simulink model "IndustrialMicrogrid"  (R2025a)
settings: Solver=FixedStepAuto  StartTime=0.0  StopTime=8  FixedStep=Ts  RelTol=1e-3
PostLoadFcn:
  | IndustrialMicrogridInputData
  | GfmGridFormingConverterInputParameters
model workspace (MAT data in the model file):
  caseNum = 2
undefined symbols (not defined in the file): base, BESS, DiscIntNeverNeededParam, grid, Grid, gridInverter, machine, microgrid, PV, PVInverter, PVTransformer, scrFactorRg, scrFactorXg, transformer, Transition_and_Dispatch_ControlModeType, Ts
libraries: ee_lib x126, fl_lib x91, eeGeneralControl x73, nesl_utility x50, nesl_utility_internal x46, simulink x30, eeTransforms x11, eeSinusoidalMeasurementV2 x5, eeTotalHarmonicDistorsion x4, slpidlib x3, simulink_extras x2, eePowerMeasurement x2
(part 8 of 12)

== system IndustrialMicrogrid/MG1 Primary Substation/BESS and Controller/BESS/Filter & Sensor ==
  Current Sensor (Three-Phase) : ee_lib/Sensors & Transducers/Current Sensor (Three-Phase)
  Electrical Reference1 : fl_lib/Electrical/Electrical Elements/Electrical Reference
  Low-Pass Filter (Discrete or Continuous)1 : eeGeneralControl/Low-Pass Filter (Discrete or Continuous)  K=1  T=1/(200*gridInverter.frequency)  B=inf  A=-inf  init_option=Specify as parameter  x0=0  Ts=gridInverter.controller.VoltageControlSampleTime
  Low-Pass Filter (Discrete or Continuous)2 : eeGeneralControl/Low-Pass Filter (Discrete or Continuous)  K=1  T=1/(200*gridInverter.frequency)  B=inf  A=-inf  init_option=Specify as parameter  x0=0  Ts=gridInverter.controller.VoltageControlSampleTime
  Neutral Port (Three-Phase) : ee_lib/Connectors & References/Neutral Port (Three-Phase)  G_parasitic=1e-12 1/Ohm
      settings: InternalSimscapePortConfiguration="{\"Bottom\":[],\"Left\":[{\"id\":\"N\",\"label\":\"~\",\"type\":\"foundation.electrical.three_phase\"}],\"Right\":[{\"id\":\"n\",\"label\":\"n\",\"type\":\"foundation.electrical.electrical\"}],\"Top\":[]}"
  PS-Simulink Converter : nesl_utility/PS-Simulink Converter  PhysicalDomain=network_engine_domain  SubClassName=ps_output  LeftPortType=input  RightPortType=output  PseudoPeriodic=off  Frequencies=[]  VectorFormat=inherit  Unit=inherit  AffineConversion=off
  PS-Simulink Converter1 : nesl_utility/PS-Simulink Converter  PhysicalDomain=network_engine_domain  SubClassName=ps_output  LeftPortType=input  RightPortType=output  PseudoPeriodic=off  Frequencies=[]  VectorFormat=inherit  Unit=inherit  AffineConversion=off
  Phase Voltage Sensor (Three-Phase) : ee_lib/Sensors & Transducers/Phase Voltage Sensor (Three-Phase)
  RLC (Three-Phase) : ee_lib/Passive/RLC Assemblies/RLC (Three-Phase)  port_option=ee.enum.threePhasePort.composite  component_structure=ee.enum.rlc.structure.SeriesRL  R=gridInverter.lineResistance Ohm  L=gridInverter.L*10 H  C=1e-6 F  R_parasitic=0 Ohm  G_parasitic=0 1/Ohm  IL_specify=off  IL_priority=High  IL=[0, 0, 0] A  IL_nominal_specify=off  IL_nominal_value=1  IL_nominal_unit=A  VC_specify=off  VC_priority=High  VC=[0, 0, 0] V  VC_nominal_specify=off  VC_nominal_value=1  VC_nominal_unit=V
      settings: InternalSimscapePortConfiguration="{\"Bottom\":[],\"Left\":[{\"id\":\"N1\",\"label\":\"~1\",\"type\":\"foundation.electrical.three_phase\"}],\"Right\":[{\"id\":\"N2\",\"label\":\"~2\",\"type\":\"foundation.electrical.three_phase\"}],\"Top\":[]}"
  Inabc : PMIOPort  Side=Left
  Opabc : PMIOPort  Port=2  Side=Right
  Iabc : Outport
  Vabc : Outport  Port=2
  wires:
  PS-Simulink Converter1/1 -> Low-Pass Filter (Discrete or Continuous)1/1
  Low-Pass Filter (Discrete or Continuous)2/1 -> Iabc/1
  PS-Simulink Converter/1 -> Low-Pass Filter (Discrete or Continuous)2/1
  Low-Pass Filter (Discrete or Continuous)1/1 -> Vabc/1
  connections:
  Electrical Reference1/LConn1 -- Neutral Port (Three-Phase)/RConn1
  PS-Simulink Converter1/LConn1 -- Phase Voltage Sensor (Three-Phase)/RConn1
  Current Sensor (Three-Phase)/RConn2 -- RLC (Three-Phase)/LConn1
  Neutral Port (Three-Phase)/LConn1 -- Phase Voltage Sensor (Three-Phase)/RConn2
  Current Sensor (Three-Phase)/LConn1 -- Inabc/RConn1
  PS-Simulink Converter/LConn1 -- Current Sensor (Three-Phase)/RConn1
  Phase Voltage Sensor (Three-Phase)/LConn1 -- Opabc/RConn1 -- RLC (Three-Phase)/RConn1

== system IndustrialMicrogrid/MG1 Primary Substation/BESS and Controller/BESS/Grid-Forming Converter Control ==
  Pref : Inport
  Qref : Inport  Port=2
  Vref : Inport  Port=3
  Fref : Inport  Port=4
  CntrlFlag : Inport  Port=5
  BlackStart : Inport  Port=6
  Igabc : Inport  Port=7
  Vgabc : Inport  Port=8
  Current Limiting : Subsystem
  Grid Voltage Reactive Power Support : Subsystem
  Measurement : Subsystem
      mask Display: image('$imagefile'); % Use "Edit Image" on toolstrip to change.
  Power Control : Subsystem
  VoltageCurrentControl : Subsystem
      settings: PortSchema="{\"entries\":[{\"content\":{\"sides\":[{\"content\":{\"connectorIds\":[\"In1\",\"In2\",\"In3\"]},\"type\":\"ConnectorPlacement.EquallySpacedRectSide\",\"uuid\":\"0bf15a12-7bc0-47e4-89bd-435769673763\"},{\"content\":{\"connectorIds\":[\"Out1\"],\"side\":\"RIGHT\"},\"type\":\"ConnectorPlacement.EquallySpacedRectSide\",\"uuid\":\"44a15d74-8878-4ec6-abe4-be0b1b609519\"},{\"content\":{\"connectorIds\":[\"In4\"],\"side\":\"TOP\"},\"type\":\"ConnectorPlacement.EquallySpacedRectSide\",\"uuid\":\"7a96781e-5638-4b2a-8101-d5785aae9f0f\"}]},\"type\":\"ConnectorPlacement.EquallySpacedConnector\",\"uuid\":\"4b3373ad-cf20-4175-894e-3bd1604dd0ce\"}],\"packageUris\":[\"http://schema.mathworks.com/mf0/Connector/R2020b\"],\"version\":\"1.0\"}"
  mabc : Outport
  Pmeas : Outport  Port=2
  Qmeas : Outport  Port=3
  fmeas : Outport  Port=4
  wires:
  VoltageCurrentControl/1(mabc) -> mabc/1
  Vgabc/1 -> Measurement/1(Vgabcc)
  Igabc/1 -> Measurement/2(Igabc)
  Measurement/2(Pmeas) -> Pmeas/1
  Measurement/3(Qmeas) -> Qmeas/1
  Measurement/1(measure) -> Current Limiting/1(measure), VoltageCurrentControl/4(measure), Power Control/1(measure), Grid Voltage Reactive Power Support/1(measure)
  Power Control/3(angle) -> Measurement/3(Angle)
  Power Control/1(reactiveControl) -> Current Limiting/2(reactiveControl)
  Power Control/2(activeControl) -> VoltageCurrentControl/2(activeControl)
  Current Limiting/1(currentLimiting) -> VoltageCurrentControl/1(currentLimiting)
  Qref/1 -> Grid Voltage Reactive Power Support/3(QrefInput)
  Pref/1 -> Grid Voltage Reactive Power Support/2(PrefInput)
  Grid Voltage Reactive Power Support/1(Pref) -> Power Control/2(Pref)
  Grid Voltage Reactive Power Support/2(Qref) -> Power Control/3(Qref)
  Measurement/4(fmeas) -> fmeas/1
  Fref/1 -> Power Control/5(Fref)
  Vref/1 -> Power Control/4(Vref)
  CntrlFlag/1 -> Power Control/6(CntrlFlag)
  BlackStart/1 -> VoltageCurrentControl/3(BlackStart)

== system IndustrialMicrogrid/MG1 Primary Substation/BESS and Controller/BESS/Subsystem ==
  PQref : Inport
  Demux : Demux  Outputs=2
  Low-Pass Filter (Discrete or Continuous) : eeGeneralControl/Low-Pass Filter (Discrete or Continuous)  K=1  T=5e-2  B=inf  A=-inf  init_option=Inherited from block input  x0=0  Ts=-1
  Low-Pass Filter (Discrete or Continuous)1 : eeGeneralControl/Low-Pass Filter (Discrete or Continuous)  K=1  T=5e-2  B=inf  A=-inf  init_option=Inherited from block input  x0=0  Ts=-1
  Unit Delay1 : UnitDelay  InitialCondition=1  SampleTime=Ts  HasFrameUpgradeWarning=on
  Unit Delay2 : UnitDelay  InitialCondition=1  SampleTime=Ts  HasFrameUpgradeWarning=on
  Pref : Outport
  Qref : Outport  Port=2
  wires:
  Demux/1 -> Unit Delay2/1  "Pref"
  Low-Pass Filter (Discrete or Continuous)/1 -> Pref/1
  Low-Pass Filter (Discrete or Continuous)1/1 -> Qref/1
  Demux/2 -> Unit Delay1/1  "Qref"
  PQref/1 -> Demux/1
  Unit Delay2/1 -> Low-Pass Filter (Discrete or Continuous)/1
  Unit Delay1/1 -> Low-Pass Filter (Discrete or Continuous)1/1

== system IndustrialMicrogrid/MG1 Primary Substation/BESS and Controller/BESS/Subsystem1 ==
  In1 : Inport
  Constant : Constant
  Constant1 : Constant  Value=0
  Switch : Switch  Criteria=u2 > Threshold  Threshold=0.5  SaturateOnIntegerOverflow=off  InputSameDT=off
  Out1 : Outport
  wires:
  Constant1/1 -> Switch/1
  Constant/1 -> Switch/3
  Switch/1 -> Out1/1
  In1/1 -> Switch/2

== system IndustrialMicrogrid/MG1 Primary Substation/BESS and Controller/BESS/Subsystem2 ==
  In1 : Inport
  In2 : Inport  Port=2
  AND : Logic  IconShape=distinctive  AllPortsSameDT=off  OutDataTypeStr=boolean
  Constant : Constant  Value=0
  Delay : Delay  DelayLength=microgrid.controller2BlackStartDelay  SampleTime=Ts*20000
  NOT : Logic  Operator=NOT  IconShape=distinctive  AllPortsSameDT=off  OutDataTypeStr=boolean
  Simulink-PS Converter : nesl_utility/Simulink-PS Converter  PhysicalDomain=network_engine_domain  SubClassName=ps_input  LeftPortType=input  RightPortType=output  PseudoPeriodic=off  Frequencies=[]  NoiseDistribution=none  NoiseParameters=[]  Unit=1  AffineConversion=off  FilteringAndDerivatives=provide  SimscapeFilterOrder=1  InputFilterTimeConstant=0.001  UdotUserProvided=0
  Switch : Switch  Criteria=u2 > Threshold  Threshold=0.5  SaturateOnIntegerOverflow=off  InputSameDT=off
  output : PMIOPort  Side=Right
  wires:
  AND/1 -> Switch/2
  Switch/1 -> Simulink-PS Converter/1
  In2/1 -> Switch/3
  In1/1 -> AND/1, Delay/1
  NOT/1 -> AND/2
  Constant/1 -> Switch/1
  Delay/1 -> NOT/1
  connections:
  Simulink-PS Converter/RConn1 -- output/RConn1

== system IndustrialMicrogrid/MG1 Primary Substation/BESS and Controller/BESS output filter and transformer1/Transformer 1 kV//13.8 kV ==
  "Transformer " : ee_lib/Passive/Transformers/Two-Winding Transformer (Three-Phase)  SRated=base.power*1e3 A*V  FRated=gridInverter.frequency Hz  Winding1Connection=ee.enum.windingconnection.Yg  VRated1=transformer.primaryRMSVoltage V  Winding2Connection=ee.enum.windingconnection.delta1  VRated2=transformer.secondaryRMSVoltage V  CoreType=ee.enum.coretype.threelimb  pu_Rw1=transformer.PrimaryResistancePU%*scrFactorRg  pu_Rw2=transformer.SecondaryResistancePU%*scrFactorRg  leakage_reactance_option=ee.enum.transformer_leakage.include  pu_Xl1=transformer.PrimaryReactancePU%*scrFactorXg  pu_Xl2=transformer.SecondaryReactancePU%*scrFactorXg  magnetizing_resistance_option=ee.enum.transformer_magnetizingResistance.exclude  pu_Rm=500  magnetizing_reactance_option=ee.enum.transformer_magnetizingReactance.exclude  saturation_option=ee.enum.transformer_saturation.exclude  pu_Xm=500  current_data=[0, .002, 1, 2]  magnetic_flux_data=[0, 1.2, 1.5, 1.51]  pu_X0=transformer.ZeroSequenceReactancePU%*scrFactorXg*1.1  i1_specify=on  i1_priority=None  i1=[0, 0, 0] A  i1_nominal_specify=off  i1_nominal_value=1  i1_nominal_unit=A  i2_specify=on  i2_priority=None  i2=[0, 0, 0] A  i2_nominal_specify=off  i2_nominal_value=1  i2_nominal_unit=A  phi_specify=off  phi_priority=None  phi=[0, 0, 0]  phi_nominal_specify=off  phi_nominal_value=1  phi_nominal_unit=1  power_dissipated_specify=off  power_dissipated_priority=None  power_dissipated=0 W  power_dissipated_nominal_specify=off  power_dissipated_nominal_value=1  power_dissipated_nominal_unit=W
      settings: InternalSimscapePortConfiguration="{\"Bottom\":[],\"Left\":[{\"id\":\"N1\",\"label\":\"~1\",\"type\":\"foundation.electrical.three_phase\"}],\"Right\":[{\"id\":\"N2\",\"label\":\"~2\",\"type\":\"foundation.electrical.three_phase\"}],\"Top\":[]}"
  ABC1 : PMIOPort  Side=Left
  ABC2 : PMIOPort  Port=2  Side=Right
  connections:
  "Transformer "/RConn1 -- ABC2/RConn1
  ABC1/RConn1 -- "Transformer "/LConn1

== system IndustrialMicrogrid/MG1 Primary Substation/Microgrid Controller/Microgrid Supervisory Control/Transition and Dispatch Control/On.Black_Start ==
  blackStartComplete : Inport
  blackStartEnable : Inport  Port=2
  " Demux " : Demux  Outputs=1
  " SFunction " : S-Function  Tag=Stateflow S-Function 6  FunctionName=sf_sfun  PortCounts=[2 3]  SFunctionDeploymentMode=off  EnableBusSupport=off
  " Terminator " : Terminator
  blackStartStatus : Outport
  blackStart : Outport  Port=2
  wires:
  blackStartComplete/1 -> " SFunction "/1
  blackStartEnable/1 -> " SFunction "/2
  " SFunction "/2 -> blackStartStatus/1  "blackStartStatus"
  " SFunction "/3 -> blackStart/1  "blackStart"
  " Demux "/1 -> " Terminator "/1
  " SFunction "/1 -> " Demux "/1

== system IndustrialMicrogrid/MG1 Primary Substation/Microgrid Controller/Microgrid Supervisory Control/Transition and Dispatch Control/On.Planned_Islanding ==
  PlannedIslanding : Inport
  " Demux " : Demux  Outputs=1
  " SFunction " : S-Function  Tag=Stateflow S-Function 14  FunctionName=sf_sfun  PortCounts=[1 5]  SFunctionDeploymentMode=off  EnableBusSupport=off
  " Terminator " : Terminator
  PCC : Outport
  plannedIslanding : Outport  Port=2
  plannedIslandingDispatch : Outport  Port=3
  plannedIslandingStatus : Outport  Port=4
  wires:
  PlannedIslanding/1 -> " SFunction "/1
  " SFunction "/2 -> PCC/1  "PCC"
  " SFunction "/3 -> plannedIslanding/1  "plannedIslanding"
  " SFunction "/4 -> plannedIslandingDispatch/1  "plannedIslandingDispatch"
  " SFunction "/5 -> plannedIslandingStatus/1  "plannedIslandingStatus"
  " Demux "/1 -> " Terminator "/1
  " SFunction "/1 -> " Demux "/1

== system IndustrialMicrogrid/MG1 Primary Substation/Microgrid Controller/Microgrid Supervisory Control/Transition and Dispatch Control/On.Resynchronization ==
  Resync : Inport
  " Demux " : Demux  Outputs=1
  " SFunction " : S-Function  Tag=Stateflow S-Function 15  FunctionName=sf_sfun  PortCounts=[1 5]  SFunctionDeploymentMode=off  EnableBusSupport=off
  " Terminator " : Terminator
  PCC : Outport
  resync : Outport  Port=2
  resyncStatus : Outport  Port=3
  resyncDispatch : Outport  Port=4
  wires:
  Resync/1 -> " SFunction "/1
  " SFunction "/2 -> PCC/1  "PCC"
  " SFunction "/3 -> resync/1  "resync"
  " SFunction "/4 -> resyncStatus/1  "resyncStatus"
  " SFunction "/5 -> resyncDispatch/1  "resyncDispatch"
  " Demux "/1 -> " Terminator "/1
  " SFunction "/1 -> " Demux "/1

== system IndustrialMicrogrid/MG1 Primary Substation/Microgrid Controller/Microgrid Supervisory Control/Transition and Dispatch Control/On.Steady_State_Grid_Connected ==
  resyncDispatch : Inport
  " Demux " : Demux  Outputs=1
  " SFunction " : S-Function  Tag=Stateflow S-Function 16  FunctionName=sf_sfun  PortCounts=[1 2]  SFunctionDeploymentMode=off  EnableBusSupport=off
  " Terminator " : Terminator
  emergencyDispatch : Outport
  wires:
  resyncDispatch/1 -> " SFunction "/1
  " SFunction "/2 -> emergencyDispatch/1  "emergencyDispatch"
  " Demux "/1 -> " Terminator "/1
  " SFunction "/1 -> " Demux "/1

== system IndustrialMicrogrid/MG1 Primary Substation/Microgrid Controller/Microgrid Supervisory Control/Transition and Dispatch Control/On.Steady_State_Islanded ==
  plannedIslandingDispatch : Inport
  " Demux " : Demux  Outputs=1
  " SFunction " : S-Function  Tag=Stateflow S-Function 17  FunctionName=sf_sfun  PortCounts=[1 2]  SFunctionDeploymentMode=off  EnableBusSupport=off
  " Terminator " : Terminator
  emergencyDispatch : Outport
  wires:
  plannedIslandingDispatch/1 -> " SFunction "/1
  " SFunction "/2 -> emergencyDispatch/1  "emergencyDispatch"
  " Demux "/1 -> " Terminator "/1
  " SFunction "/1 -> " Demux "/1

== system IndustrialMicrogrid/MG1 Primary Substation/Microgrid Controller/Microgrid Supervisory Control/Transition and Dispatch Control/On.Unplanned_Islanding ==
  " Demux " : Demux  Outputs=1
  " Ground " : Ground
  " SFunction " : S-Function  Tag=Stateflow S-Function 18  FunctionName=sf_sfun  PortCounts=[1 3]  SFunctionDeploymentMode=off  EnableBusSupport=off
  " Terminator " : Terminator
  PCC : Outport
  emergencyDispatch : Outport  Port=2
  wires:
  " SFunction "/2 -> PCC/1  "PCC"
  " SFunction "/3 -> emergencyDispatch/1  "emergencyDispatch"
  " Ground "/1 -> " SFunction "/1
  " Demux "/1 -> " Terminator "/1
  " SFunction "/1 -> " Demux "/1

== system IndustrialMicrogrid/MG2 PV Plant/(500KWp PV)/PV Inverter A2/PV & Inverter ==
  note: Calculated PV power output
  note: Measured PV current
  note: Perturb & Observe method for maximum power point (MPP) tracking of PV array
  note: DC bus voltage reference (which is the MPP voltage)
  Solar insolation : Inport
  reference : Inport  Port=2
  Average-Inverter : ee_lib/Semiconductors & Converters/Converters/Average-Value Voltage Source Converter (Three-Phase)  port_option=ee.enum.threePhasePort.composite  frequency_option=ee.enum.converters.frequency.variable  input_option=ee.enum.converters.inputOption.ModWave  FRated=60 Hz  losses_parameterization=ee.enum.converters.losses.fixed  Pfixed=1 W  ks=0.01  kc1=1.7 V  kc2=0.01 Ohm  Ploss_vect=[100, 800, 1870, 3250, 4900] W  Irms_vect=[10, 100, 200, 300, 400] A  Vdc_nom=300 V  thermal_mass=30000 J/K  temperature_specify=off  temperature_priority=High  temperature=298.15 K  temperature_nominal_specify=off  temperature_nominal_value=1  temperature_nominal_unit=K
      settings: InternalSimscapePortConfiguration="{\"Bottom\":[],\"Left\":[{\"id\":\"ModWave\",\"label\":\"ModWave\",\"type\":\"input\"},{\"id\":\"N\",\"label\":\"~\",\"type\":\"foundation.electrical.three_phase\"}],\"Right\":[{\"id\":\"p\",\"label\":\"+\",\"type\":\"foundation.electrical.electrical\"},{\"id\":\"n\",\"label\":\"-\",\"type\":\"foundation.electrical.electrical\"}],\"Top\":[]}"
  Current Sensor : fl_lib/Electrical/Electrical Sensors/Current Sensor
  DC- Capacitor : fl_lib/Electrical/Electrical Elements/Capacitor  c=PVInverter.c F  r=1e-6 Ohm  g=0 1/Ohm  i_specify=off  i_priority=None  i=0 A  i_nominal_specify=off  i_nominal_value=1  i_nominal_unit=A  v_specify=off  v_priority=None  v=6560*.5 V  v_nominal_specify=off  v_nominal_value=1  v_nominal_unit=V  vc_specify=on  vc_priority=None  vc=PVInverter.Vdc V  vc_nominal_specify=off  vc_nominal_value=1  vc_nominal_unit=V
  ERef1 : fl_lib/Electrical/Electrical Elements/Electrical Reference
  Low-Pass Filter (Discrete or Continuous) : eeGeneralControl/Low-Pass Filter (Discrete or Continuous)  K=1  T=0.2  B=inf  A=-inf  init_option=Inherited from block input  x0=0  Ts=-1
  Low-Pass Filter (Discrete or Continuous)1 : eeGeneralControl/Low-Pass Filter (Discrete or Continuous)  K=1  T=0.2  B=inf  A=-inf  init_option=Inherited from block input  x0=0  Ts=-1
  Measurement1 : Subsystem
  Measurement2 : Subsystem
  P&O MPP : Subsystem
  PS-Simulink Converter : nesl_utility/PS-Simulink Converter  PhysicalDomain=network_engine_domain  SubClassName=ps_output  LeftPortType=input  RightPortType=output  PseudoPeriodic=off  Frequencies=[]  VectorFormat=inherit  Unit=inherit  AffineConversion=off
  PS-Simulink Converter1 : nesl_utility/PS-Simulink Converter  PhysicalDomain=network_engine_domain  SubClassName=ps_output  LeftPortType=input  RightPortType=output  PseudoPeriodic=off  Frequencies=[]  VectorFormat=inherit  Unit=inherit  AffineConversion=off
  PV Array : ee_lib/Sources/Solar Cell  prm=3  Isc=3.8 A  Voc=0.586 V  Is=PV.solarCellDiodeSaturationCurrent A  Is2=0 A  Iph=PV.solarCellSolarGeneratedCurrentAM A  Ir0=1000 W/m^2  ec=PV.solarCellQualityFactorI  N2=PV.solarCellQualityFactorJ  Rs=PV.solarCellSeriesResistance Ohm  Rp=PV.solarCellParallelResistance Ohm  N_series=PV.panelNSeriesCellPanel*PV.arrayNseriesPanelsPerString  N_parallel=PV.PanelNParallelStringsPanel*PV.arrayNParallelStrings  TIPH1=PV.solarCellTempCofficient 1/K  EG=PV.solarCellEg eV  TXIS1=PV.solarCellTemparatureExponentIs1  TXIS2=PV.solarCellTemparatureExponentIs2  TRS1=PV.solarCellTemparatureExponentRs  TRP1=PV.solarCellTemparatureExponentRp  Tmeas=PV.solarCellMeasurementTemperature degC  TFIXED=PV.solarCellDeviceTemperature degC  thermal_mass=100 J/K  initial_temperature=25 degC
  Product2 : Product
  Simulink-PS Converter1 : nesl_utility/Simulink-PS Converter  PhysicalDomain=network_engine_domain  SubClassName=ps_input  LeftPortType=input  RightPortType=output  PseudoPeriodic=off  Frequencies=[]  NoiseDistribution=none  NoiseParameters=[]  Unit=1  AffineConversion=off  FilteringAndDerivatives=provide  SimscapeFilterOrder=1  InputFilterTimeConstant=0.001  UdotUserProvided=0
  Simulink-PS Converter2 : nesl_utility/Simulink-PS Converter  PhysicalDomain=network_engine_domain  SubClassName=ps_input  LeftPortType=input  RightPortType=output  PseudoPeriodic=off  Frequencies=[]  NoiseDistribution=none  NoiseParameters=[]  Unit=1  AffineConversion=off  FilteringAndDerivatives=provide  SimscapeFilterOrder=1  InputFilterTimeConstant=0.001  UdotUserProvided=0
  Voltage Sensor : fl_lib/Electrical/Electrical Sensors/Voltage Sensor
  Conn1 : PMIOPort  Side=Right
  Out Bus Element4 : Outport  PortName=PV_plant1  Element=Vdc_ref
  Out Bus Element : Outport  PortName=PV_plant1  Element=Pref1
  Out Bus Element3 : Outport  PortName=PV_plant1  Element=Vdc_measured
  Out Bus Element1 : Outport  PortName=PV_plant1  Element=ipv
  wires:
  Low-Pass Filter (Discrete or Continuous)1/1 -> Product2/2
  Low-Pass Filter (Discrete or Continuous)/1 -> [Vdc]
  Measurement2/1(Out1) -> [ipv]
  Measurement1/1(Out1) -> Low-Pass Filter (Discrete or Continuous)/1
  [Vdc] -> P&O MPP/2(Input)
  P&O MPP/1(Vmpp) -> Out Bus Element4/1
  Product2/1 -> Out Bus Element/1, P&O MPP/1(In1)
  reference/1 -> Simulink-PS Converter2/1
  [Vdc] -> Product2/1
  PS-Simulink Converter/1 -> Out Bus Element3/1, Measurement1/1(u)
  [ipv] -> Low-Pass Filter (Discrete or Continuous)1/1
  Solar insolation/1 -> Simulink-PS Converter1/1
  PS-Simulink Converter1/1 -> Out Bus Element1/1, Measurement2/1(u)
  connections:
  PV Array/RConn1 -- ERef1/LConn1 -- DC- Capacitor/RConn1 -- Average-Inverter/RConn2 -- Voltage Sensor/RConn2
  Simulink-PS Converter1/RConn1 -- PV Array/LConn1
  PS-Simulink Converter1/LConn1 -- Current Sensor/RConn1
  Conn1/RConn1 -- Average-Inverter/LConn2
  PV Array/LConn2 -- Current Sensor/LConn1
  Average-Inverter/LConn1 -- Simulink-PS Converter2/RConn1
  Voltage Sensor/LConn1 -- Current Sensor/RConn2 -- Average-Inverter/RConn1 -- DC- Capacitor/LConn1
  PS-Simulink Converter/LConn1 -- Voltage Sensor/RConn1

== system IndustrialMicrogrid/MG2 PV Plant/(500KWp PV)/PV Inverter A2/PV Controller ==
  note: DQ/abc Transformation
  In Bus Element17 : Inport  PortName=PV_plant1  Element=Pref1
  In Bus Element18 : Inport  PortName=PV_plant1  Element=Vdc_measured
  In Bus Element19 : Inport  PortName=PV_plant1  Element=Vdc_ref
  In Bus Element5 : Inport  Port=2  PortName=ipv1  Element=1
  In Bus Element4 : Inport  Port=3  PortName=LVRT
  In Bus Element3 : Inport  Port=4  PortName=Vbus  Element=Vd
  In Bus Element1 : Inport  Port=4  PortName=Vbus  Element=Vd
  In Bus Element2 : Inport  Port=4  PortName=Vbus  Element=Vq
  In Bus Element6 : Inport  Port=4  PortName=Vbus  Element=Theta
  In Bus Element7 : Inport  Port=4  PortName=Vbus  Element=Theta
  Q_ref : Inport  Port=5
  Current_controller : Subsystem
  DC voltage controller & current reference : Subsystem
  Demux1 : Demux  Outputs=3
  Inverse Park Transform1 : eeTransforms/Inverse Park Transform  AxisAlignment=Q-axis  PowerInvariant=off
  Park Transform1 : eeTransforms/Park Transform  AxisAlignment=Q-axis  PowerInvariant=off
  Terminator1 : Terminator
  Unit Delay2 : UnitDelay  SampleTime=Ts  HasFrameUpgradeWarning=on
  m_abc : Outport
  wires:
  Q_ref/1 -> DC voltage controller & current reference/1(Q_ref)
  DC voltage controller & current reference/2(id_ref) -> [id_ref]
  DC voltage controller & current reference/1(iq_ref) -> [iq_ref]
  In Bus Element19/1 -> DC voltage controller & current reference/5(PV_vdc)
  In Bus Element18/1 -> DC voltage controller & current reference/4(PV_Mpp_vdc)
  In Bus Element17/1 -> DC voltage controller & current reference/3(P_pv)
  In Bus Element4/1 -> DC voltage controller & current reference/6(LVRT.iq)
  In Bus Element1/1 -> DC voltage controller & current reference/2(Vmag)
  In Bus Element5/1 -> Park Transform1/1
  [ipvd] -> Current_controller/2(ipvd)
  In Bus Element7/1 -> Inverse Park Transform1/2
  In Bus Element6/1 -> Park Transform1/2
  [ipvq] -> Current_controller/4(iq)
  [iq_ref] -> Current_controller/3(iqref)
  In Bus Element3/1 -> Current_controller/5(Vd)
  [id_ref] -> Current_controller/1(id-ref)
  Park Transform1/1 -> Demux1/1
  [mdqo] -> Inverse Park Transform1/1
  Demux1/3 -> Terminator1/1
  Demux1/1 -> [ipvd]
  Unit Delay2/1 -> m_abc/1
  Demux1/2 -> [ipvq]
  Inverse Park Transform1/1 -> Unit Delay2/1
  Current_controller/1(Refrence_mdq0) -> [mdqo]
  In Bus Element2/1 -> Current_controller/6(Vq)

== system IndustrialMicrogrid/MG2 Power Center/Diesel Generator/Governor and Prime Mover /Governor ==
  pu_velocity : Inport
  1/T_G : Gain  Gain=1/T_G
  1/droop : Gain  Gain=1/(droop_percentage/100)
  Delta load setpoint : Sum  Inputs=+-|
  Delta speed : Sum  Inputs=-+|
  Discrete-Time Integrator1 : DiscreteIntegrator  InitialCondition=pu_torque0  SampleTime=-1  ICPrevOutput=DiscIntNeverNeededParam  ICPrevScaledInput=DiscIntNeverNeededParam
  Load_setpoint : Constant  Value=pu_load_reference_setpoint
  Speed_ref : Constant  Value=pu_speed_reference
  Subtract : Sum  Inputs=|+-
  delta_y : Outport  VectorParamsAs1DForOutWhenUnconnected=off
  wires:
  Speed_ref/1 -> Delta speed/1
  Delta speed/1 -> 1/droop/1
  Load_setpoint/1 -> Delta load setpoint/1
  pu_velocity/1 -> Delta speed/2
  1/droop/1 -> Delta load setpoint/2
  Delta load setpoint/1 -> Subtract/1
  Subtract/1 -> 1/T_G/1
  1/T_G/1 -> Discrete-Time Integrator1/1
  Discrete-Time Integrator1/1 -> delta_y/1, Subtract/2

== system IndustrialMicrogrid/MG2 Power Center/Diesel Generator/Governor and Prime Mover /Non-reheat turbine ==
  delta_y : Inport
  1/T_CH : Gain  Gain=1/T_CH
  Discrete-Time Integrator1 : DiscreteIntegrator  InitialCondition=pu_torque0  SampleTime=-1  ICPrevOutput=DiscIntNeverNeededParam  ICPrevScaledInput=DiscIntNeverNeededParam
  Sum : Sum  Inputs=|+-
  torque : Outport  VectorParamsAs1DForOutWhenUnconnected=off
  wires:
  delta_y/1 -> Sum/1
  Sum/1 -> 1/T_CH/1
  1/T_CH/1 -> Discrete-Time Integrator1/1
  Discrete-Time Integrator1/1 -> Sum/2, torque/1

== system IndustrialMicrogrid/MG2 Primary Substation/BESS and Controller/BESS/Filter & Sensor ==
  Current Sensor (Three-Phase) : ee_lib/Sensors & Transducers/Current Sensor (Three-Phase)
  Electrical Reference1 : fl_lib/Electrical/Electrical Elements/Electrical Reference
  Low-Pass Filter (Discrete or Continuous)1 : eeGeneralControl/Low-Pass Filter (Discrete or Continuous)  K=1  T=1/(200*gridInverter.frequency)  B=inf  A=-inf  init_option=Specify as parameter  x0=0  Ts=gridInverter.controller.VoltageControlSampleTime
  Low-Pass Filter (Discrete or Continuous)2 : eeGeneralControl/Low-Pass Filter (Discrete or Continuous)  K=1  T=1/(200*gridInverter.frequency)  B=inf  A=-inf  init_option=Specify as parameter  x0=0  Ts=gridInverter.controller.VoltageControlSampleTime
  Neutral Port (Three-Phase) : ee_lib/Connectors & References/Neutral Port (Three-Phase)  G_parasitic=1e-12 1/Ohm
      settings: InternalSimscapePortConfiguration="{\"Bottom\":[],\"Left\":[{\"id\":\"N\",\"label\":\"~\",\"type\":\"foundation.electrical.three_phase\"}],\"Right\":[{\"id\":\"n\",\"label\":\"n\",\"type\":\"foundation.electrical.electrical\"}],\"Top\":[]}"
  PS-Simulink Converter : nesl_utility/PS-Simulink Converter  PhysicalDomain=network_engine_domain  SubClassName=ps_output  LeftPortType=input  RightPortType=output  PseudoPeriodic=off  Frequencies=[]  VectorFormat=inherit  Unit=inherit  AffineConversion=off
  PS-Simulink Converter1 : nesl_utility/PS-Simulink Converter  PhysicalDomain=network_engine_domain  SubClassName=ps_output  LeftPortType=input  RightPortType=output  PseudoPeriodic=off  Frequencies=[]  VectorFormat=inherit  Unit=inherit  AffineConversion=off
  Phase Voltage Sensor (Three-Phase) : ee_lib/Sensors & Transducers/Phase Voltage Sensor (Three-Phase)
  RLC (Three-Phase) : ee_lib/Passive/RLC Assemblies/RLC (Three-Phase)  port_option=ee.enum.threePhasePort.composite  component_structure=ee.enum.rlc.structure.SeriesRL  R=gridInverter.lineResistance*2 Ohm  L=gridInverter.L*10 H  C=1e-6 F  R_parasitic=0 Ohm  G_parasitic=0 1/Ohm  IL_specify=on  IL_priority=None  IL=[0, 0, 0] A  IL_nominal_specify=off  IL_nominal_value=1  IL_nominal_unit=A  VC_specify=off  VC_priority=High  VC=[0, 0, 0] V  VC_nominal_specify=off  VC_nominal_value=1  VC_nominal_unit=V
      settings: InternalSimscapePortConfiguration="{\"Bottom\":[],\"Left\":[{\"id\":\"N1\",\"label\":\"~1\",\"type\":\"foundation.electrical.three_phase\"}],\"Right\":[{\"id\":\"N2\",\"label\":\"~2\",\"type\":\"foundation.electrical.three_phase\"}],\"Top\":[]}"
  Inabc : PMIOPort  Side=Left
  Opabc : PMIOPort  Port=2  Side=Right
  Iabc : Outport
  Vabc : Outport  Port=2
  wires:
  PS-Simulink Converter1/1 -> Low-Pass Filter (Discrete or Continuous)1/1
  Low-Pass Filter (Discrete or Continuous)2/1 -> Iabc/1
  PS-Simulink Converter/1 -> Low-Pass Filter (Discrete or Continuous)2/1
  Low-Pass Filter (Discrete or Continuous)1/1 -> Vabc/1
  connections:
  Electrical Reference1/LConn1 -- Neutral Port (Three-Phase)/RConn1
  PS-Simulink Converter1/LConn1 -- Phase Voltage Sensor (Three-Phase)/RConn1
  Current Sensor (Three-Phase)/RConn2 -- RLC (Three-Phase)/LConn1
  Neutral Port (Three-Phase)/LConn1 -- Phase Voltage Sensor (Three-Phase)/RConn2
  Current Sensor (Three-Phase)/LConn1 -- Inabc/RConn1
  PS-Simulink Converter/LConn1 -- Current Sensor (Three-Phase)/RConn1
  Phase Voltage Sensor (Three-Phase)/LConn1 -- Opabc/RConn1 -- RLC (Three-Phase)/RConn1

== system IndustrialMicrogrid/MG2 Primary Substation/BESS and Controller/BESS/Grid-Forming Converter Control ==
  Pref : Inport
  Qref : Inport  Port=2
  Vref : Inport  Port=3
  Fref : Inport  Port=4
  CntrlFlag : Inport  Port=5
  BlackStart : Inport  Port=6
  Igabc : Inport  Port=7
  Vgabc : Inport  Port=8
  Current Limiting : Subsystem
  Grid Voltage Reactive Power Support : Subsystem
  Measurement : Subsystem
      mask Display: image('$imagefile'); % Use "Edit Image" on toolstrip to change.
  Power Control : Subsystem
  VoltageCurrentControl : Subsystem
      settings: PortSchema="{\"entries\":[{\"content\":{\"sides\":[{\"content\":{\"connectorIds\":[\"In1\",\"In2\",\"In3\"]},\"type\":\"ConnectorPlacement.EquallySpacedRectSide\",\"uuid\":\"0bf15a12-7bc0-47e4-89bd-435769673763\"},{\"content\":{\"connectorIds\":[\"Out1\"],\"side\":\"RIGHT\"},\"type\":\"ConnectorPlacement.EquallySpacedRectSide\",\"uuid\":\"44a15d74-8878-4ec6-abe4-be0b1b609519\"},{\"content\":{\"connectorIds\":[\"In4\"],\"side\":\"TOP\"},\"type\":\"ConnectorPlacement.EquallySpacedRectSide\",\"uuid\":\"7a96781e-5638-4b2a-8101-d5785aae9f0f\"}]},\"type\":\"ConnectorPlacement.EquallySpacedConnector\",\"uuid\":\"4b3373ad-cf20-4175-894e-3bd1604dd0ce\"}],\"packageUris\":[\"http://schema.mathworks.com/mf0/Connector/R2020b\"],\"version\":\"1.0\"}"
  mabc : Outport
  Pmeas : Outport  Port=2
  Qmeas : Outport  Port=3
  fmeas : Outport  Port=4
  wires:
  VoltageCurrentControl/1(mabc) -> mabc/1
  Vgabc/1 -> Measurement/1(Vgabcc)
  Igabc/1 -> Measurement/2(Igabc)
  Measurement/2(Pmeas) -> Pmeas/1
  Measurement/3(Qmeas) -> Qmeas/1
  Measurement/1(measure) -> Current Limiting/1(measure), VoltageCurrentControl/4(measure), Power Control/1(measure), Grid Voltage Reactive Power Support/1(measure)
  Power Control/3(angle) -> Measurement/3(Angle)
  Power Control/1(reactiveControl) -> Current Limiting/2(reactiveControl)
  Power Control/2(activeControl) -> VoltageCurrentControl/2(activeControl)
  Current Limiting/1(currentLimiting) -> VoltageCurrentControl/1(currentLimiting)
  Qref/1 -> Grid Voltage Reactive Power Support/3(QrefInput)
  Pref/1 -> Grid Voltage Reactive Power Support/2(PrefInput)
  Grid Voltage Reactive Power Support/1(Pref) -> Power Control/2(Pref)
  Grid Voltage Reactive Power Support/2(Qref) -> Power Control/3(Qref)
  Measurement/4(fmeas) -> fmeas/1
  Fref/1 -> Power Control/5(Fref)
  Vref/1 -> Power Control/4(Vref)
  CntrlFlag/1 -> Power Control/6(CntrlFlag)
  BlackStart/1 -> VoltageCurrentControl/3(BlackStart)

== system IndustrialMicrogrid/MG2 Primary Substation/BESS and Controller/BESS/Subsystem ==
  PQref : Inport
  Demux : Demux  Outputs=2
  Low-Pass Filter (Discrete or Continuous) : eeGeneralControl/Low-Pass Filter (Discrete or Continuous)  K=1  T=5e-2  B=inf  A=-inf  init_option=Inherited from block input  x0=0  Ts=-1
  Low-Pass Filter (Discrete or Continuous)1 : eeGeneralControl/Low-Pass Filter (Discrete or Continuous)  K=1  T=5e-2  B=inf  A=-inf  init_option=Inherited from block input  x0=0  Ts=-1
  Unit Delay1 : UnitDelay  InitialCondition=1  SampleTime=Ts  HasFrameUpgradeWarning=on
  Unit Delay2 : UnitDelay  InitialCondition=1  SampleTime=Ts  HasFrameUpgradeWarning=on
  Pref : Outport
  Qref : Outport  Port=2
  wires:
  Demux/1 -> Unit Delay2/1  "Pref"
  Low-Pass Filter (Discrete or Continuous)/1 -> Pref/1
  Low-Pass Filter (Discrete or Continuous)1/1 -> Qref/1
  Demux/2 -> Unit Delay1/1  "Qref"
  PQref/1 -> Demux/1
  Unit Delay2/1 -> Low-Pass Filter (Discrete or Continuous)/1
  Unit Delay1/1 -> Low-Pass Filter (Discrete or Continuous)1/1

== system IndustrialMicrogrid/MG2 Primary Substation/BESS and Controller/BESS/Subsystem1 ==
  In1 : Inport
  Constant : Constant
  Constant1 : Constant  Value=0
  Switch : Switch  Criteria=u2 > Threshold  Threshold=0.5  SaturateOnIntegerOverflow=off  InputSameDT=off
  Out1 : Outport
  wires:
  Constant1/1 -> Switch/1
  Constant/1 -> Switch/3
  Switch/1 -> Out1/1
  In1/1 -> Switch/2

== system IndustrialMicrogrid/MG2 Primary Substation/BESS and Controller/BESS/Subsystem2 ==
  In1 : Inport
  In2 : Inport  Port=2
  AND : Logic  IconShape=distinctive  AllPortsSameDT=off  OutDataTypeStr=boolean
  Constant : Constant  Value=0
  Delay : Delay  DelayLength=microgrid.controller2BlackStartDelay  SampleTime=Ts*20000
  NOT : Logic  Operator=NOT  IconShape=distinctive  AllPortsSameDT=off  OutDataTypeStr=boolean
  Simulink-PS Converter : nesl_utility/Simulink-PS Converter  PhysicalDomain=network_engine_domain  SubClassName=ps_input  LeftPortType=input  RightPortType=output  PseudoPeriodic=off  Frequencies=[]  NoiseDistribution=none  NoiseParameters=[]  Unit=1  AffineConversion=off  FilteringAndDerivatives=provide  SimscapeFilterOrder=1  InputFilterTimeConstant=0.001  UdotUserProvided=0
  Switch : Switch  Criteria=u2 > Threshold  Threshold=0.5  SaturateOnIntegerOverflow=off  InputSameDT=off
  output : PMIOPort  Side=Right
  wires:
  AND/1 -> Switch/2
  Switch/1 -> Simulink-PS Converter/1
  In2/1 -> Switch/3
  In1/1 -> AND/1, Delay/1
  NOT/1 -> AND/2
  Constant/1 -> Switch/1
  Delay/1 -> NOT/1
  connections:
  Simulink-PS Converter/RConn1 -- output/RConn1

== system IndustrialMicrogrid/MG2 Primary Substation/BESS and Controller/BESS output filter and transformer1/Transformer 1 kV//13.8 kV ==
  "Transformer " : ee_lib/Passive/Transformers/Two-Winding Transformer (Three-Phase)  SRated=base.power*1e3 A*V  FRated=gridInverter.frequency Hz  Winding1Connection=ee.enum.windingconnection.Yg  VRated1=transformer.primaryRMSVoltage V  Winding2Connection=ee.enum.windingconnection.delta1  VRated2=transformer.secondaryRMSVoltage V  CoreType=ee.enum.coretype.threelimb  pu_Rw1=transformer.PrimaryResistancePU%*scrFactorRg  pu_Rw2=transformer.SecondaryResistancePU%*scrFactorRg  leakage_reactance_option=ee.enum.transformer_leakage.include  pu_Xl1=transformer.PrimaryReactancePU%*scrFactorXg  pu_Xl2=transformer.SecondaryReactancePU%*scrFactorXg  magnetizing_resistance_option=ee.enum.transformer_magnetizingResistance.exclude  pu_Rm=500  magnetizing_reactance_option=ee.enum.transformer_magnetizingReactance.exclude  saturation_option=ee.enum.transformer_saturation.exclude  pu_Xm=500  current_data=[0, .002, 1, 2]  magnetic_flux_data=[0, 1.2, 1.5, 1.51]  pu_X0=transformer.ZeroSequenceReactancePU%*scrFactorXg*1.1  i1_specify=on  i1_priority=None  i1=[0, 0, 0] A  i1_nominal_specify=off  i1_nominal_value=1  i1_nominal_unit=A  i2_specify=on  i2_priority=None  i2=[0, 0, 0] A  i2_nominal_specify=off  i2_nominal_value=1  i2_nominal_unit=A  phi_specify=off  phi_priority=None  phi=[0, 0, 0]  phi_nominal_specify=off  phi_nominal_value=1  phi_nominal_unit=1  power_dissipated_specify=off  power_dissipated_priority=None  power_dissipated=0 W  power_dissipated_nominal_specify=off  power_dissipated_nominal_value=1  power_dissipated_nominal_unit=W
      settings: InternalSimscapePortConfiguration="{\"Bottom\":[],\"Left\":[{\"id\":\"N1\",\"label\":\"~1\",\"type\":\"foundation.electrical.three_phase\"}],\"Right\":[{\"id\":\"N2\",\"label\":\"~2\",\"type\":\"foundation.electrical.three_phase\"}],\"Top\":[]}"
  ABC1 : PMIOPort  Side=Left
  ABC2 : PMIOPort  Port=2  Side=Right
  connections:
  "Transformer "/RConn1 -- ABC2/RConn1
  ABC1/RConn1 -- "Transformer "/LConn1

== system IndustrialMicrogrid/MG2 Primary Substation/Microgrid Controller/Microgrid Supervisory Control/Transition and Dispatch Control/On.Black_Start ==
  blackStartComplete : Inport
  blackStartEnable : Inport  Port=2
  " Demux " : Demux  Outputs=1
  " SFunction " : S-Function  Tag=Stateflow S-Function 11  FunctionName=sf_sfun  PortCounts=[2 3]  SFunctionDeploymentMode=off  EnableBusSupport=off
  " Terminator " : Terminator
  blackStartStatus : Outport
  blackStart : Outport  Port=2
  wires:
  blackStartComplete/1 -> " SFunction "/1
  blackStartEnable/1 -> " SFunction "/2
  " SFunction "/2 -> blackStartStatus/1  "blackStartStatus"
  " SFunction "/3 -> blackStart/1  "blackStart"
  " Demux "/1 -> " Terminator "/1
  " SFunction "/1 -> " Demux "/1

== system IndustrialMicrogrid/MG2 Primary Substation/Microgrid Controller/Microgrid Supervisory Control/Transition and Dispatch Control/On.Planned_Islanding ==
  PlannedIslanding : Inport
  " Demux " : Demux  Outputs=1
  " SFunction " : S-Function  Tag=Stateflow S-Function 1  FunctionName=sf_sfun  PortCounts=[1 5]  SFunctionDeploymentMode=off  EnableBusSupport=off
  " Terminator " : Terminator
  PCC : Outport
  plannedIslanding : Outport  Port=2
  plannedIslandingDispatch : Outport  Port=3
  plannedIslandingStatus : Outport  Port=4
  wires:
  PlannedIslanding/1 -> " SFunction "/1
  " SFunction "/2 -> PCC/1  "PCC"
  " SFunction "/3 -> plannedIslanding/1  "plannedIslanding"
  " SFunction "/4 -> plannedIslandingDispatch/1  "plannedIslandingDispatch"
  " SFunction "/5 -> plannedIslandingStatus/1  "plannedIslandingStatus"
  " Demux "/1 -> " Terminator "/1
  " SFunction "/1 -> " Demux "/1

== system IndustrialMicrogrid/MG2 Primary Substation/Microgrid Controller/Microgrid Supervisory Control/Transition and Dispatch Control/On.Resynchronization ==
  Resync : Inport
  " Demux " : Demux  Outputs=1
  " SFunction " : S-Function  Tag=Stateflow S-Function 7  FunctionName=sf_sfun  PortCounts=[1 5]  SFunctionDeploymentMode=off  EnableBusSupport=off
  " Terminator " : Terminator
  PCC : Outport
  resync : Outport  Port=2
  resyncStatus : Outport  Port=3
  resyncDispatch : Outport  Port=4
  wires:
  Resync/1 -> " SFunction "/1
  " SFunction "/2 -> PCC/1  "PCC"
  " SFunction "/3 -> resync/1  "resync"
  " SFunction "/4 -> resyncStatus/1  "resyncStatus"
  " SFunction "/5 -> resyncDispatch/1  "resyncDispatch"
  " Demux "/1 -> " Terminator "/1
  " SFunction "/1 -> " Demux "/1

== system IndustrialMicrogrid/MG2 Primary Substation/Microgrid Controller/Microgrid Supervisory Control/Transition and Dispatch Control/On.Steady_State_Grid_Connected ==
  resyncDispatch : Inport
  " Demux " : Demux  Outputs=1
  " SFunction " : S-Function  Tag=Stateflow S-Function 8  FunctionName=sf_sfun  PortCounts=[1 2]  SFunctionDeploymentMode=off  EnableBusSupport=off
  " Terminator " : Terminator
  emergencyDispatch : Outport
  wires:
  resyncDispatch/1 -> " SFunction "/1
  " SFunction "/2 -> emergencyDispatch/1  "emergencyDispatch"
  " Demux "/1 -> " Terminator "/1
  " SFunction "/1 -> " Demux "/1

== system IndustrialMicrogrid/MG2 Primary Substation/Microgrid Controller/Microgrid Supervisory Control/Transition and Dispatch Control/On.Steady_State_Islanded ==
  plannedIslandingDispatch : Inport
  " Demux " : Demux  Outputs=1
  " SFunction " : S-Function  Tag=Stateflow S-Function 9  FunctionName=sf_sfun  PortCounts=[1 2]  SFunctionDeploymentMode=off  EnableBusSupport=off
  " Terminator " : Terminator
  emergencyDispatch : Outport
  wires:
  plannedIslandingDispatch/1 -> " SFunction "/1
  " SFunction "/2 -> emergencyDispatch/1  "emergencyDispatch"
  " Demux "/1 -> " Terminator "/1
  " SFunction "/1 -> " Demux "/1

== system IndustrialMicrogrid/MG2 Primary Substation/Microgrid Controller/Microgrid Supervisory Control/Transition and Dispatch Control/On.Unplanned_Islanding ==
  " Demux " : Demux  Outputs=1
  " Ground " : Ground
  " SFunction " : S-Function  Tag=Stateflow S-Function 10  FunctionName=sf_sfun  PortCounts=[1 3]  SFunctionDeploymentMode=off  EnableBusSupport=off
  " Terminator " : Terminator
  PCC : Outport
  emergencyDispatch : Outport  Port=2
  wires:
  " SFunction "/2 -> PCC/1  "PCC"
  " SFunction "/3 -> emergencyDispatch/1  "emergencyDispatch"
  " Ground "/1 -> " SFunction "/1
  " Demux "/1 -> " Terminator "/1
  " SFunction "/1 -> " Demux "/1

== system IndustrialMicrogrid/Operator Room/MG1/Measurements and Visualizations /Mode Selection ==
  Mode : Inport
  Mode-0 : simulink/Logic and Bit Operations/Compare To Constant  relop===  const=Transition_and_Dispatch_ControlModeType.None  OutDataTypeStr=boolean
  Mode-1 : simulink/Logic and Bit Operations/Compare To Constant  relop===  const=Transition_and_Dispatch_ControlModeType.Steady_State_Islanded  OutDataTypeStr=boolean
  Mode-2 : simulink/Logic and Bit Operations/Compare To Constant  relop===  const=Transition_and_Dispatch_ControlModeType.Resynchronization  OutDataTypeStr=boolean
  Mode-3 : simulink/Logic and Bit Operations/Compare To Constant  relop===  const=Transition_and_Dispatch_ControlModeType.Steady_State_Grid_Connected  OutDataTypeStr=boolean
  Mode-4 : simulink/Logic and Bit Operations/Compare To Constant  relop===  const=Transition_and_Dispatch_ControlModeType.Planned_Islanding  OutDataTypeStr=boolean
  Mode-5 : simulink/Logic and Bit Operations/Compare To Constant  relop===  const=Transition_and_Dispatch_ControlModeType.Black_Start  OutDataTypeStr=boolean
  Mode-6 : simulink/Logic and Bit Operations/Compare To Constant  relop===  const=Transition_and_Dispatch_ControlModeType.Unplanned_Islanding  OutDataTypeStr=boolean
  Scope : Scope  NumInputPorts=7
      settings: ActiveDisplayYMinimum=-0.125  ActiveDisplayYMaximum=1.125  DataLoggingVariableName=ScopeData3
  wires:
  Mode/1 -> Mode-5/1, Mode-6/1, Mode-4/1, Mode-3/1, Mode-2/1, Mode-1/1, Mode-0/1
  Mode-5/1 -> Scope/6  "Mode-5"
  Mode-0/1 -> Scope/1  "Mode-0"
  Mode-1/1 -> Scope/2  "Mode-1"
  Mode-2/1 -> Scope/3  "Mode-2"
  Mode-3/1 -> Scope/4  "Mode-3"
  Mode-6/1 -> Scope/7  "Mode-6"
  Mode-4/1 -> Scope/5  "Mode-4"

== system IndustrialMicrogrid/Operator Room/MG2/Measurements and Visualizations/Mode Selection ==
  Mode : Inport
  Mode-0 : simulink/Logic and Bit Operations/Compare To Constant  relop===  const=Transition_and_Dispatch_ControlModeType.None  OutDataTypeStr=boolean
  Mode-1 : simulink/Logic and Bit Operations/Compare To Constant  relop===  const=Transition_and_Dispatch_ControlModeType.Steady_State_Islanded  OutDataTypeStr=boolean
  Mode-2 : simulink/Logic and Bit Operations/Compare To Constant  relop===  const=Transition_and_Dispatch_ControlModeType.Resynchronization  OutDataTypeStr=boolean
  Mode-3 : simulink/Logic and Bit Operations/Compare To Constant  relop===  const=Transition_and_Dispatch_ControlModeType.Steady_State_Grid_Connected  OutDataTypeStr=boolean
  Mode-4 : simulink/Logic and Bit Operations/Compare To Constant  relop===  const=Transition_and_Dispatch_ControlModeType.Planned_Islanding  OutDataTypeStr=boolean
  Mode-5 : simulink/Logic and Bit Operations/Compare To Constant  relop===  const=Transition_and_Dispatch_ControlModeType.Black_Start  OutDataTypeStr=boolean
  Mode-6 : simulink/Logic and Bit Operations/Compare To Constant  relop===  const=Transition_and_Dispatch_ControlModeType.Unplanned_Islanding  OutDataTypeStr=boolean
  Scope : Scope  NumInputPorts=7
      settings: ActiveDisplayYMinimum=-0.125  ActiveDisplayYMaximum=1.125  DataLoggingVariableName=ScopeData3
  wires:
  Mode/1 -> Mode-5/1, Mode-6/1, Mode-4/1, Mode-3/1, Mode-2/1, Mode-1/1, Mode-0/1
  Mode-5/1 -> Scope/6  "Mode-5"
  Mode-0/1 -> Scope/1  "Mode-0"
  Mode-1/1 -> Scope/2  "Mode-1"
  Mode-2/1 -> Scope/3  "Mode-2"
  Mode-3/1 -> Scope/4  "Mode-3"
  Mode-6/1 -> Scope/7  "Mode-6"
  Mode-4/1 -> Scope/5  "Mode-4"

== system IndustrialMicrogrid/MG1 Primary Substation/BESS and Controller/BESS/Grid-Forming Converter Control/Current Limiting ==
  In Bus Element : Inport  PortName=measure  Element=Igd
  In Bus Element1 : Inport  PortName=measure  Element=Igq
  In Bus Element2 : Inport  Port=2  PortName=reactiveControl  Element=Vmd
  In Bus Element4 : Inport  Port=2  PortName=reactiveControl  Element=Vmq
  CurrentLimitingMethod : Subsystem  Variant=on  VariantControlMode=label  VariantControl=Choice  LabelModeActiveChoice=virimp
  Subtract : Sum  Inputs=+-
  Subtract1 : Sum  Inputs=-+
  Out Bus Element : Outport  PortName=currentLimiting  Element=Vmd
  Out Bus Element1 : Outport  PortName=currentLimiting  Element=Vmq
  Out Bus Element2 : Outport  PortName=currentLimiting  Element=Idmax
  Out Bus Element3 : Outport  PortName=currentLimiting  Element=Iqmax
  wires:
  In Bus Element2/1 -> Subtract/1
  In Bus Element1/1 -> CurrentLimitingMethod/2(Igq)
  In Bus Element4/1 -> Subtract1/2
  Subtract/1 -> Out Bus Element/1
  Subtract1/1 -> Out Bus Element1/1
  CurrentLimitingMethod/4(Iqmax) -> Out Bus Element3/1
  In Bus Element/1 -> CurrentLimitingMethod/1(Igd)  "Q"
  CurrentLimitingMethod/3(Idmax) -> Out Bus Element2/1
  CurrentLimitingMethod/1(delVd) -> Subtract/2
  CurrentLimitingMethod/2(delVq) -> Subtract1/1

== system IndustrialMicrogrid/MG1 Primary Substation/BESS and Controller/BESS/Grid-Forming Converter Control/Grid Voltage Reactive Power Support ==
  In Bus Element1 : Inport  PortName=measure  Element=Vgd
  In Bus Element3 : Inport  PortName=measure  Element=Vgq
  In Bus Element2 : Inport  PortName=measure  Element=Igd
  In Bus Element4 : Inport  PortName=measure  Element=Igq
  PrefInput : Inport  Port=2
  QrefInput : Inport  Port=3
  Modifying Active Power Reference : Subsystem
  Modifying Reactive Power Reference : Subsystem
  Pref : Outport
  Qref : Outport  Port=2
  wires:
  Modifying Active Power Reference/1(Pref) -> Modifying Reactive Power Reference/4(Pref)
  PrefInput/1 -> Modifying Active Power Reference/1(PrefInput)
  In Bus Element2/1 -> Modifying Active Power Reference/3(Igd)
  In Bus Element4/1 -> Modifying Active Power Reference/4(Igq)
  In Bus Element1/1 -> Modifying Reactive Power Reference/1(Vgd), Modifying Active Power Reference/2(Vd)
  In Bus Element3/1 -> Modifying Reactive Power Reference/2(Vgq)
  QrefInput/1 -> Modifying Reactive Power Reference/3(Qref)
  Modifying Reactive Power Reference/1(PrefNew) -> Pref/1
  Modifying Reactive Power Reference/2(QrefNew) -> Qref/1

== system IndustrialMicrogrid/MG1 Primary Substation/BESS and Controller/BESS/Grid-Forming Converter Control/Measurement ==
  Vgabcc : Inport
  Igabc : Inport  Port=2
  Angle : Inport  Port=3
  Frequency Measurement : Subsystem
  Gain1 : Gain  Gain=1/power
  Gain2 : Gain  Gain=1/power
  Gain3 : Gain  Gain=1/(girdLineVoltage*sqrt(2/3))
  Gain4 : Gain  Gain=1/(girdLineVoltage*sqrt(2/3))
  Gain5 : Gain  Gain=1/(power/(sqrt(3)*girdLineVoltage)*sqrt(2))
  Gain6 : Gain  Gain=1/(power/(sqrt(3)*girdLineVoltage)*sqrt(2))
  Power Measurement (Three-Phase) : eePowerMeasurement/Power Measurement (Three-Phase)  LabelModeActiveChoice=Discrete  F=powerFreq  K=[1]  Seq=Positive  Ts=measSampleTime
  abc2dq : Subsystem
  Out Bus Element : Outport  PortName=measure  Element=P
  Out Bus Element1 : Outport  PortName=measure  Element=Q
  Out Bus Element2 : Outport  PortName=measure  Element=Vgd
  Out Bus Element3 : Outport  PortName=measure  Element=Vgq
  Out Bus Element4 : Outport  PortName=measure  Element=Igd
  Out Bus Element5 : Outport  PortName=measure  Element=Igq
  Out Bus Element6 : Outport  PortName=measure  Element=fgrid
  Pmeas : Outport  Port=2
  Qmeas : Outport  Port=3
  fmeas : Outport  Port=4
  wires:
  Vgabcc/1 -> abc2dq/3(Vgabc), Frequency Measurement/1(Vabc), Power Measurement (Three-Phase)/1  "Vabc"
  Angle/1 -> abc2dq/2(Angle)
  Power Measurement (Three-Phase)/1 -> Gain2/1
  Igabc/1 -> abc2dq/1(Igabc), Power Measurement (Three-Phase)/2  "Iabc"
  Power Measurement (Three-Phase)/2 -> Gain1/1
  Gain2/1 -> Pmeas/1, Out Bus Element/1  "Pmeas"
  Gain1/1 -> Qmeas/1, Out Bus Element1/1  "Qmeas"
  abc2dq/1(Vgd) -> Gain4/1
  abc2dq/2(Vgq) -> Gain3/1
  abc2dq/3(Igd) -> Gain5/1
  abc2dq/4(Igq) -> Gain6/1
  Gain3/1 -> Out Bus Element3/1  "Vgq"
  Gain4/1 -> Out Bus Element2/1  "Vgd"
  Gain5/1 -> Out Bus Element4/1  "Igd"
  Gain6/1 -> Out Bus Element5/1  "Igq"
  Frequency Measurement/1(freq) -> Out Bus Element6/1, fmeas/1
